simulink model "tut5"  (R2024a)
settings: Solver=FixedStepDiscrete  StartTime=0.0  StopTime=50  FixedStep=.02  RelTol=1e-3
values from neighbouring files (symbols this model uses):
  ActiveMode =     [matlab.mat]
  Command =     [matlab.mat]
  Fan_Input_Modes =     [matlab.mat]
  Fan_Modes =     [matlab.mat]
  RequestedMode =     [matlab.mat]
  State =     [matlab.mat]
libraries: spsStairGeneratorLib x3
settings Model: Creator=User  LastModifiedBy=User

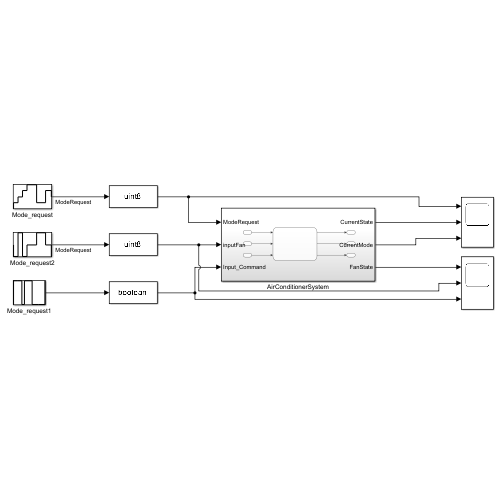
[thumbnail: Simulink's stored preview of the top-level diagram]
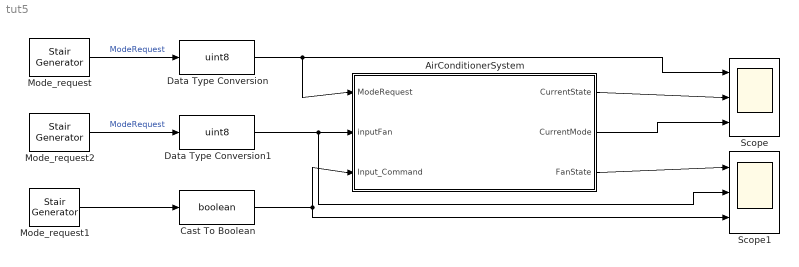
== system tut5 ==
  AirConditionerSystem : Subsystem
  Cast To Boolean : DataTypeConversion  OutDataTypeStr=boolean  SaturateOnIntegerOverflow=off  RndMeth=Floor
  Data Type Conversion : DataTypeConversion  OutDataTypeStr=uint8  SaturateOnIntegerOverflow=off  RndMeth=Floor
  Data Type Conversion1 : DataTypeConversion  OutDataTypeStr=uint8  SaturateOnIntegerOverflow=off  RndMeth=Floor
  Mode_request : spsStairGeneratorLib/Stair Generator  t=[0, 2.5, 7.5, 12.5,17.5,28,38,44]  e=[0, 1, 2, 3,4,1,3,2]  Ts=0
  Mode_request1 : spsStairGeneratorLib/Stair Generator  t=[0, 4, 9, 15,18,28,37,45]  e=[0, 1, 1, 0,1,0,0,1]  Ts=0
  Mode_request2 : spsStairGeneratorLib/Stair Generator  t=[0, 2.5, 7.5, 12.5,17.5,28,38,44]  e=[2, 1, 3, 1,2,3,2,1]  Ts=0
  Scope : Scope  NumInputPorts=3
  Scope1 : Scope  NumInputPorts=3
  wires:
  Mode_request/1 -> Data Type Conversion/1  "ModeRequest"
  Mode_request1/1 -> Cast To Boolean/1
  AirConditionerSystem/1(CurrentState) -> Scope/2
  AirConditionerSystem/2(CurrentMode) -> Scope/3
  Cast To Boolean/1 -> Scope1/3, AirConditionerSystem/3(Input_Command)
  Data Type Conversion/1 -> Scope/1, AirConditionerSystem/1(ModeRequest)
  Mode_request2/1 -> Data Type Conversion1/1  "ModeRequest"
  Data Type Conversion1/1 -> Scope1/2, AirConditionerSystem/2(inputFan)
  AirConditionerSystem/3(FanState) -> Scope1/1

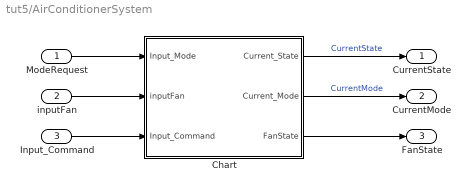
== system tut5/AirConditionerSystem ==
  ModeRequest : Inport  OutDataTypeStr=uint8
  inputFan : Inport  Port=2  OutDataTypeStr=uint8
  Input_Command : Inport  Port=3  OutDataTypeStr=boolean
  Chart : Stateflow chart  TreatAsAtomicUnit=on
  CurrentState : Outport  OutDataTypeStr=boolean
  CurrentMode : Outport  Port=2  OutDataTypeStr=uint8
  FanState : Outport  Port=3  OutDataTypeStr=uint8
  wires:
  inputFan/1 -> Chart/2(inputFan)
  Chart/1(Current_State) -> CurrentState/1  "CurrentState"
  Chart/3(FanState) -> FanState/1
  Input_Command/1 -> Chart/3(Input_Command)
  Chart/2(Current_Mode) -> CurrentMode/1  "CurrentMode"
  ModeRequest/1 -> Chart/1(Input_Mode)

== stateflow chart tut5/AirConditionerSystem/Chart ==
  state Main [parallel]
    settings: executionOrder=1
    state OFF
      en:Current_State=boolean(State.OFF);
      en:Current_Mode=uint8(ActiveMode.Off);
      state Off1
      state Off2
      (default) -> Off1
      Off1 -> Off2
    state ON
      en:Current_State=boolean(State.ON);
      state Hot1
        en:Current_Mode=uint8(ActiveMode.Hot);
      state Cold1
        en:Current_Mode=uint8(ActiveMode.Cold);
      state Wet1
        en:Current_Mode=uint8(ActiveMode.Wet);
      state Dry1
        en:Current_Mode=uint8(ActiveMode.Dry);
      (default) -> Cold1
      Cold1 -> (junction 145) : [Input_Mode ~=RequestedMode.Cold]
      Hot1 -> (junction 145) : [Input_Mode ~= RequestedMode.Hot]
      (junction 145) -> (junction 151)
      (junction 158) -> Cold1 [order 1] : [Input_Mode ==RequestedMode.Cold]
      (junction 154) -> Hot1 [order 1] : [Input_Mode == RequestedMode.Hot]
      (junction 151) -> (junction 158) [order 2]
      (junction 151) -> (junction 154) [order 1]
      (junction 154) -> Dry1 [order 2] : [Input_Mode == RequestedMode.Dry]
      (junction 158) -> Wet1 [order 2] : [Input_Mode ~=RequestedMode.Wet]
      (junction 147) -> (junction 151)
      Dry1 -> (junction 147) : [Input_Mode ~= RequestedMode.Dry]
      Wet1 -> (junction 147) : [Input_Mode ~=RequestedMode.Wet]
    (default) -> ON
    OFF -> ON : [hasChangedTo(Input_Command,Command.ON) ]{send(Fan.GoOn);}
    ON -> OFF : [hasChangedTo(Input_Command,Command.OFF)]{send(Fan.GoOff);}
  state Fan [parallel]
    settings: executionOrder=2
    state FanOn
      state Low
        en:FanState=uint8(Fan_Modes.Low);
      state High
        en:FanState=uint8(Fan_Modes.High);
      state Mid
        en:FanState=uint8(Fan_Modes.Mid);
      (default) -> Low
      Low -> High [order 2] : [inputFan == Fan_Input_Modes.High]
      High -> Low [order 1] : [inputFan == Fan_Input_Modes.Low]
      Mid -> Low [order 2] : [inputFan == Fan_Input_Modes.Low]
      Low -> Mid [order 1] : [inputFan == Fan_Input_Modes.Mid]
      High -> Mid [order 2] : [inputFan == Fan_Input_Modes.Mid]
      Mid -> High [order 1] : [inputFan == Fan_Input_Modes.High]
    state FanOff
      en:FanState=uint8(Fan_Modes.Off);
    (default) -> FanOff
    FanOn -> FanOff : GoOff
    FanOff -> FanOn : GoOn
  data: Input_Mode input; inputFan input; Input_Command input; Current_State output boolean; Current_Mode output uint8; FanState output uint8; ActiveMode parameter; RequestedMode parameter; State parameter; Command parameter; Fan_Modes parameter; Fan_Input_Modes parameter
  events: GoOn local FUNCTION_CALL_EVENT; GoOff local FUNCTION_CALL_EVENT
